simulink model "MotorControlSim_OpenLoopPWM"  (R2025b)
settings: Solver=FixedStepAuto  FixedStep=1e-6
libraries: slpidlib x2, simulink x1
(part 2 of 2)

== system MotorControlSim_OpenLoopPWM/PMSM2/Park transform ==
  theta_e : Inport
  "ualpha, ubeta" : Inport  Port=2
  Demux : Demux  Outputs=2
  Gain : Gain  Gain=-1
  Matrix Concatenate : Concatenate  Mode=Multidimensional array  ConcatenateDimension=2
  Matrix Concatenate1 : Concatenate  Mode=Multidimensional array  ConcatenateDimension=2
  Matrix Concatenate2 : Concatenate  Mode=Multidimensional array
  Product1 : Product  Multiplication=Matrix(*)
  Sin : Trigonometry  Operator=cos
  Sin1 : Trigonometry
  ud : Outport
  uq : Outport  Port=2
  wires:
  Demux/2 -> uq/1  "uq"
  Product1/1 -> Demux/1  "ud, uq"
  Gain/1 -> Matrix Concatenate1/1
  Matrix Concatenate1/1 -> Matrix Concatenate2/2
  Sin1/1 -> Gain/1, Matrix Concatenate/2
  Matrix Concatenate2/1 -> Product1/1
  Matrix Concatenate/1 -> Matrix Concatenate2/1
  Sin/1 -> Matrix Concatenate/1, Matrix Concatenate1/2
  theta_e/1 -> Sin1/1, Sin/1
  Demux/1 -> ud/1  "ud"
  "ualpha, ubeta"/1 -> Product1/2

== system MotorControlSim_OpenLoopPWM/PMSM2/Phase voltage calculation ==
  ua0 : Inport
  ub0 : Inport  Port=2
  uc0 : Inport  Port=3
  Add : Sum  Inputs=+++
  Gain : Gain  Gain=1/3
  Subtract : Sum  Inputs=+-
  Subtract1 : Sum  Inputs=+-
  Subtract2 : Sum  Inputs=+-
  ua : Outport
  ub : Outport  Port=2
  uc : Outport  Port=3
  wires:
  uc0/1 -> Add/3, Subtract2/1
  Subtract2/1 -> uc/1
  Subtract/1 -> ua/1
  Gain/1 -> Subtract/2, Subtract1/2, Subtract2/2  "un"
  Add/1 -> Gain/1
  ua0/1 -> Subtract/1, Add/1
  ub0/1 -> Add/2, Subtract1/1
  Subtract1/1 -> ub/1

== system MotorControlSim_OpenLoopPWM/SVPWM/Common mode Injection ==
  In1 : Inport
  In2 : Inport  Port=2
  In3 : Inport  Port=3
  Add{,2..4} (4 alike) : Sum
  Gain : Gain  Gain=-1/2
  Max : MinMax  Function=max  Inputs=3
  Min : MinMax  Inputs=3
  ua,mod* : Outport
  ub,mod* : Outport  Port=2
  uc,mod* : Outport  Port=3
  wires:
  Add2/1 -> ua,mod*/1  "ua,mod*"
  Add3/1 -> ub,mod*/1  "ub,mod*"
  Min/1 -> Add/2
  Add4/1 -> uc,mod*/1  "uc,mod*"
  Add/1 -> Gain/1
  Gain/1 -> Add2/2, Add3/2, Add4/2  "u0"
  In2/1 -> Max/2, Min/2, Add3/1
  Max/1 -> Add/1
  In3/1 -> Max/3, Min/3, Add4/1
  In1/1 -> Min/1, Max/1, Add2/1

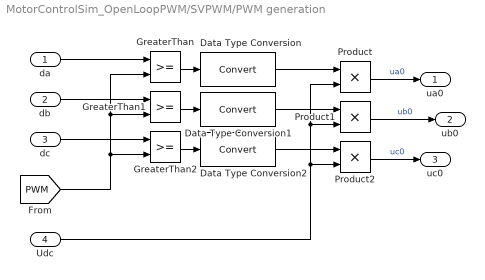
== system MotorControlSim_OpenLoopPWM/SVPWM/PWM generation ==
  da : Inport
  db : Inport  Port=2
  dc : Inport  Port=3
  Udc : Inport  Port=4
  Data Type Conversion : DataTypeConversion  SaturateOnIntegerOverflow=off  RndMeth=Floor
  Data Type Conversion1 : DataTypeConversion  SaturateOnIntegerOverflow=off  RndMeth=Floor
  Data Type Conversion2 : DataTypeConversion  SaturateOnIntegerOverflow=off  RndMeth=Floor
  GreaterThan : RelationalOperator  OutDataTypeStr=boolean  RndMeth=Simplest  InputSameDT=off
  GreaterThan1 : RelationalOperator  OutDataTypeStr=boolean  RndMeth=Simplest  InputSameDT=off
  GreaterThan2 : RelationalOperator  OutDataTypeStr=boolean  RndMeth=Simplest  InputSameDT=off
  Product : Product
  Product1 : Product
  Product2 : Product
  ua0 : Outport
  ub0 : Outport  Port=2
  uc0 : Outport  Port=3
  wires:
  Product2/1 -> uc0/1  "uc0"
  dc/1 -> GreaterThan2/1
  Udc/1 -> Product2/2, Product/2, Product1/2
  Product/1 -> ua0/1  "ua0"
  [PWM] -> GreaterThan/2, GreaterThan1/2, GreaterThan2/2
  GreaterThan/1 -> Data Type Conversion/1
  db/1 -> GreaterThan1/1
  Product1/1 -> ub0/1  "ub0"
  GreaterThan2/1 -> Data Type Conversion2/1
  GreaterThan1/1 -> Data Type Conversion1/1
  Data Type Conversion2/1 -> Product2/1
  Data Type Conversion/1 -> Product/1
  da/1 -> GreaterThan/1
  Data Type Conversion1/1 -> Product1/1
